simulink model "excercise1_2tf1"  (R2023b)
settings: Solver=VariableStepAuto  StartTime=0.0  StopTime=2  RelTol=1e-3
undefined symbols (not defined in the file): d, k, m
settings Model: Creator=elliot  LastModifiedBy=elliot

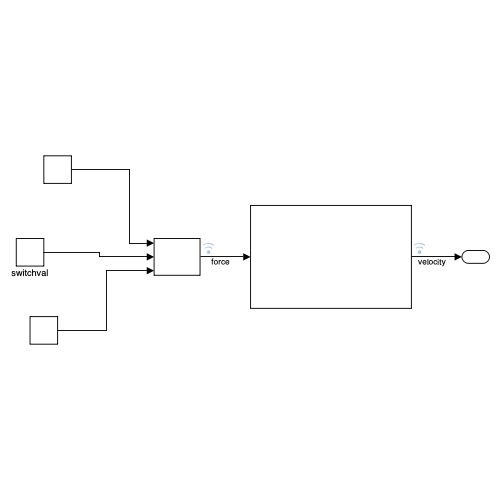
[thumbnail: Simulink's stored preview of the top-level diagram]
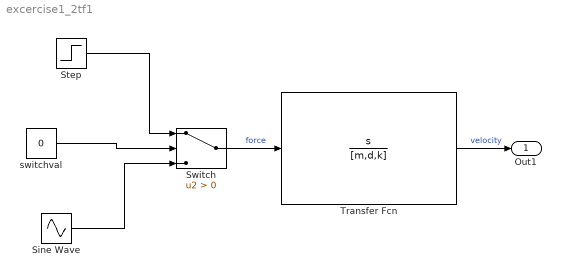
== system excercise1_2tf1 ==
  Sine Wave : Sin  Frequency=20  SampleTime=0
  Step : Step  Time=0  SampleTime=0
  Switch : Switch  Criteria=u2 > Threshold  SaturateOnIntegerOverflow=off  InputSameDT=off
  Transfer Fcn : TransferFcn  Numerator=[1, 0]  Denominator=[m,d,k]
  switchval : Constant  Value=0
  Out1 : Outport
  wires:
  Step/1 -> Switch/1
  Switch/1 -> Transfer Fcn/1  "force"
  Sine Wave/1 -> Switch/3
  Transfer Fcn/1 -> Out1/1  "velocity"
  switchval/1 -> Switch/2
